simulink model "msv_sim"  (R2021b)
settings: Solver=VariableStepAuto  StartTime=0.0  StopTime=10.0  RelTol=1e-3
undefined symbols (not defined in the file or in its folder): b, P, T_d, T_I, Vss, y
settings Model: Creator=ishaa  LastModifiedBy=ishaa

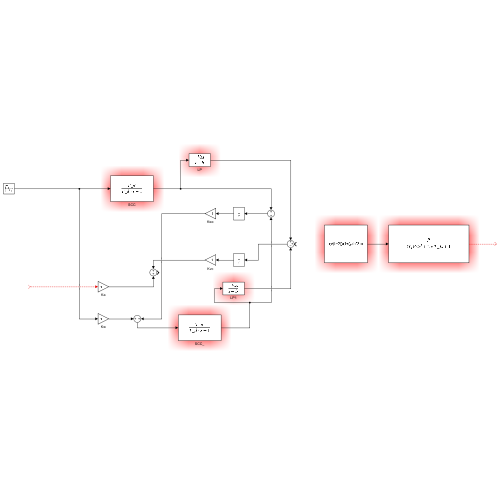
[thumbnail: Simulink's stored preview of the top-level diagram]
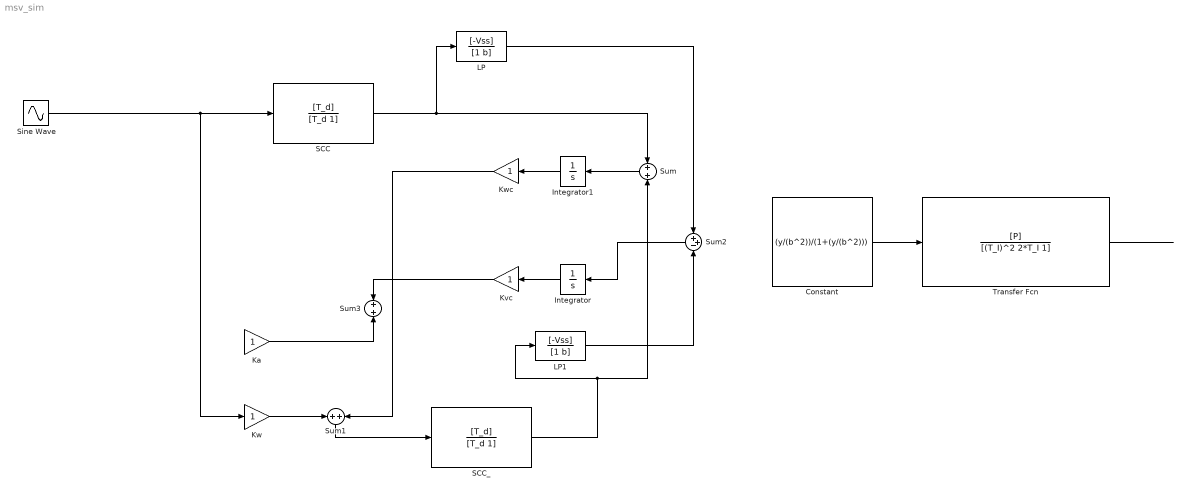
== system msv_sim ==
  Constant : Constant  Value=(y/(b^2))/(1+(y/(b^2)))
  Integrator : Integrator
  Integrator1 : Integrator
  Ka : Gain
  Kvc : Gain
  Kw : Gain
  Kwc : Gain
  LP : TransferFcn  Numerator=[-Vss]  Denominator=[1 b]
  LP1 : TransferFcn  Numerator=[-Vss]  Denominator=[1 b]
  SCC : TransferFcn  Numerator=[T_d]  Denominator=[T_d 1]
  SCC_ : TransferFcn  Numerator=[T_d]  Denominator=[T_d 1]
  Sine Wave : Sin  Frequency=0.5  SampleTime=0
  Sum : Sum
  Sum1 : Sum
  Sum2 : Sum  Inputs=++-
  Sum3 : Sum
  Transfer Fcn : TransferFcn  Numerator=[P]  Denominator=[(T_I)^2 2*T_I 1]
  wires:
  SCC/1 -> Sum/1, LP/1
  Sum/1 -> Integrator1/1
  Sum1/1 -> SCC_/1
  SCC_/1 -> LP1/1, Sum/2
  LP/1 -> Sum2/1
  Sum2/1 -> Integrator/1
  Integrator/1 -> Kvc/1
  Integrator1/1 -> Kwc/1
  Sine Wave/1 -> Kw/1, SCC/1
  ? -> Ka/1
  LP1/1 -> Sum2/3
  Kvc/1 -> Sum3/1
  Ka/1 -> Sum3/2
  Kw/1 -> Sum1/1
  Kwc/1 -> Sum1/2
  Constant/1 -> Transfer Fcn/1
  Transfer Fcn/1 -> ?
